simulink model "IRP"  (R2015a)
settings: Solver=ode1  StartTime=0.0  StopTime=Inf  FixedStep=0.001  RelTol=1e-3
PostLoadFcn:
  | , if any(exist('dsrtsu_mdlpostloadfcn', 'file') == [2, 3, 6]), try dsrtsu_mdlpostloadfcn('Execute', bdroot); catch fprintf('Error in PostLoadFcn (dsrtsu_mdlpostloadfcn) for model "%s":\n %s\n', bdroot, lasterr); end, end,
libraries: simulink x8, rtilibm x6, simulink_extras x6
(part 1 of 2)
settings Model: DSRTSU_INTERNAL_RTI_VER=460  DSRTSU_INTERNAL_RTI_TYPE=rti1005  DSRTSU_INTERNAL_RTIFPGA=50  Creator=k19p800a  LastModifiedBy=k19p800a
settings OptimizationCC: BlockReduction=off  OptimizeBlockIOStorage=off  BufferReuse=off  GlobalBufferReuse=off  ExpressionFolding=off  LocalBlockOutputs=off
settings HardwareCC: ProdIntDivRoundTo=Zero  ProdEndianess=BigEndian  ProdHWDeviceType=Generic->Custom  TargetIntDivRoundTo=Zero  TargetEndianess=BigEndian  TargetHWDeviceType=Generic->Custom
settings RTWCC: SystemTargetFile=rti1005.tlc  MakeCommand=make_rti  TemplateMakefile=rti1005.tmf  Description=dSPACE DS1005 Hardware Platform
settings STFCustomTargetCC: GenerateSampleERTMain=off  ParMdlRefBuildCompliant=on  GeneratePreprocessorConditionals=Disable all  ERTCustomFileBanners=off  SupportNonInlinedSFcns=on  SupportVariableSizeSignals=off  MATLABClassNameForMDSCustomization=Simulink.SoftwareTarget.GRTCustomization  GRTInterface=on  SystemTargetFile=rti1005.tlc
settings GRTTargetCC: CompOptLevelCompliant=off  ConcurrentExecutionCompliant=off  CombineOutputUpdateFcns=off  MatFileLogging=off  CPPClassGenCompliant=off  GRTInterface=on  ExtModeMexFile=noextcomm

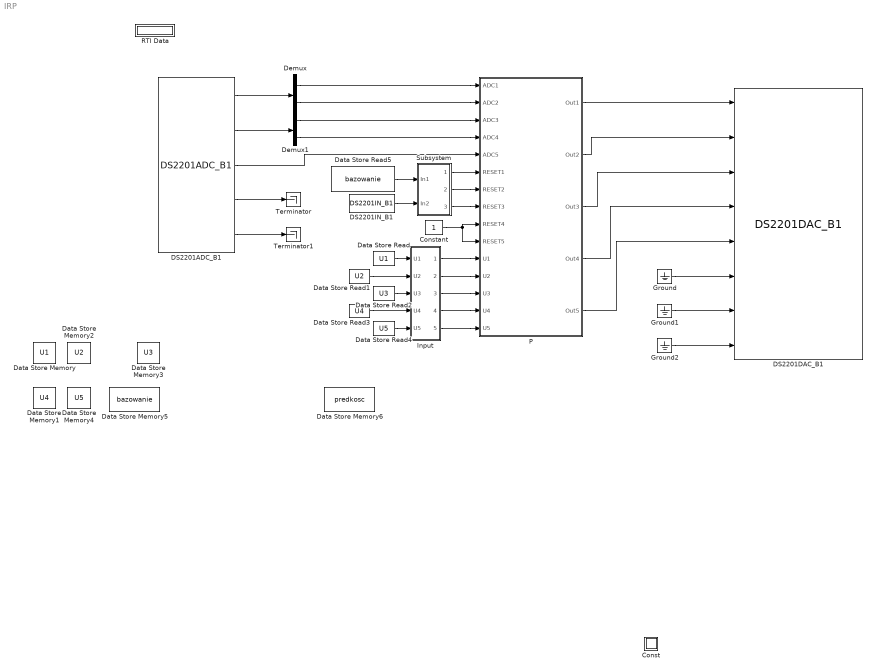
== system IRP ==
  Const : Subsystem
  Constant : Constant
  DS2201ADC_B1 : rtilibm/DS2201/DS2201ADC_B1  BoardNo=1  channelNo1=[1 2 3 4]  channelNo2=[5 6 7 8]  channelNo3=[9 10]  channelNo4=-1  channelNo5=-1  DialogFcn=gui2201adc  UnitName={'DS2201ADC_B'}  UnitValues={ 1 }  DSProperties=struct('RTI',struct('Version',uint32(1),'BlockType',struct('isSLSource',uint8(1),'isSLSink',uint8(0),'isHWSource',uint8(1),'isHWSink',uint8(0),'isSetup',uint8(0),'isInline',uint8(1),'isNonInline',uint8(0),'isInterrupt',uint8(0),'isChannelwise',uint8(0)),'IOBoardType','DS2201','UnitType','ADC','Identifier','ADCMUX','DialogType','ML','BlockSet','NONE','SlaveProcessor','NONE'))
  DS2201DAC_B1 : rtilibm/DS2201/DS2201DAC_B1  BoardNo=1  IOErrorMode=[0 0]  InitValue=[0 0 0 0 0 0 0 0]  TermMode=[1 1 1 1 1 1 1 1]  TermValue=[0 0 0 0 0 0 0 0]  DialogFcn=gui2201dac  UnitName={'DS2201DAC_B'}  UnitValues={ 1 }  DSProperties=struct('RTI',struct('Version',uint32(1),'BlockType',struct('isSLSource',uint8(0),'isSLSink',uint8(1),'isHWSource',uint8(0),'isHWSink',uint8(1),'isSetup',uint8(0),'isInline',uint8(1),'isNonInline',uint8(0),'isInterrupt',uint8(0),'isChannelwise',uint8(0)),'IOBoardType','DS2201','UnitType','DAC','Identifier','DAC','DialogType','ML','BlockSet','NONE','SlaveProcessor','NONE'))
  DS2201IN_B1 : rtilibm/DS2201/DS2201IN_B1  BoardNo=1  ChannelNos=[1 2 3 4 5]  DialogFcn=gui2201in  UnitName={ 'DS2201IN_B' }  UnitValues={ 1 }  DSProperties=struct('RTI',struct('Version',uint32(1),'BlockType',struct('isSLSource',uint8(1),'isSLSink',uint8(0),'isHWSource',uint8(1),'isHWSink',uint8(0),'isSetup',uint8(0),'isInline',uint8(1),'isNonInline',uint8(0),'isInterrupt',uint8(0),'isChannelwise',uint8(0)),'IOBoardType','DS2201','UnitType','BIT','Identifier','BITIN','DialogType','ML','BlockSet','NONE','SlaveProcessor','NONE'))
  Data Store Memory : DataStoreMemory  DataStoreName=U1  ReadBeforeWriteMsg=warning  WriteAfterWriteMsg=warning  WriteAfterReadMsg=warning
  Data Store Memory1 : DataStoreMemory  DataStoreName=U4  ReadBeforeWriteMsg=warning  WriteAfterWriteMsg=warning  WriteAfterReadMsg=warning
  Data Store Memory2 : DataStoreMemory  DataStoreName=U2  ReadBeforeWriteMsg=warning  WriteAfterWriteMsg=warning  WriteAfterReadMsg=warning
  Data Store Memory3 : DataStoreMemory  DataStoreName=U3  ReadBeforeWriteMsg=warning  WriteAfterWriteMsg=warning  WriteAfterReadMsg=warning
  Data Store Memory4 : DataStoreMemory  DataStoreName=U5  ReadBeforeWriteMsg=warning  WriteAfterWriteMsg=warning  WriteAfterReadMsg=warning
  Data Store Memory5 : DataStoreMemory  DataStoreName=bazowanie  ReadBeforeWriteMsg=warning  WriteAfterWriteMsg=warning  WriteAfterReadMsg=warning
  Data Store Memory6 : DataStoreMemory  DataStoreName=predkosc  ReadBeforeWriteMsg=warning  WriteAfterWriteMsg=warning  WriteAfterReadMsg=warning
  Data Store Read : DataStoreRead  DataStoreName=U1
  Data Store Read1 : DataStoreRead  DataStoreName=U2
  Data Store Read2 : DataStoreRead  DataStoreName=U3
  Data Store Read3 : DataStoreRead  DataStoreName=U4
  Data Store Read4 : DataStoreRead  DataStoreName=U5
  Data Store Read5 : DataStoreRead  DataStoreName=bazowanie
  Demux : Demux  Outputs=2
  Demux1 : Demux  Outputs=2
  Ground : Ground
  Ground1 : Ground
  Ground2 : Ground
  Input : Subsystem
  "P " : Subsystem
  RTI Data : Subsystem  Tag=struct('RTIDataServer',struct('RTIDataServerVs','2','RTIModelDescription','struct(''main'',''IRP'',''sub'','''',''isMp'',0)'))  LoadFcn="if exist('rtidc'), try,  rtidc('DataHostBlockClbLoad', gcbh); catch, disp(['Warning: ''LoadFcn'' for RTI Data block failed: ' lasterr]); end, end,"  mask(RTI_DATA_HOST){}
      mask help:
      | RTI Data Block.
      | This block is used by RTI to store internal model-dependent data.
      | Please keep this block on the root level of the model. Deleting this block will result in data loss.
      |
      | NEVER DELETE OR COPY THIS BLOCK!
      settings: CopyFcn="if exist('rtidc'), try,  rtidc('DataHostBlockClbCopy', gcbh); catch, disp(['Warning: ''CopyFcn'' for RTI Data block failed: ' lasterr]); end, end,"  DeleteFcn="if exist('rtidc'), try,  rtidc('DataHostBlockClbDelete', gcbh); catch, disp(['Warning: ''DeleteFcn'' for RTI Data block failed: ' lasterr]); end, end,"  ModelCloseFcn="if exist('rtidc'), try,  rtidc('DataHostBlockClbModelClose', gcbh); catch, disp(['Warning: ''ModelCloseFcn'' for RTI Data block failed: ' lasterr]); end, end,"  PreSaveFcn="if exist('rtidc'), try,  rtidc('DataHostBlockClbPreSave', gcbh); catch, disp(['Warning: ''PreSaveFcn'' for RTI Data block failed: ' lasterr]); end, end,"  PostSaveFcn="if exist('rtidc'), try,  rtidc('DataHostBlockClbPostSave', gcbh); catch, disp(['Warning: ''PostSaveFcn'' for RTI Data block failed: ' lasterr]); end, end,"  NameChangeFcn="if exist('rtidc'), try,  rtidc('DataHostBlockClbNameChange', gcbh); catch, disp(['Warning: ''NameChangeFcn'' for RTI Data block failed: ' lasterr]); end, end,"
      mask Help:
      | RTI Data Block.
      | This block is used by RTI to store internal model-dependent data.
      | Please keep this block on the root level of the model. Deleting this block will result in data loss.
      | 
      | NEVER DELETE OR COPY THIS BLOCK!
      mask Display:
      | text(0.5, 0.5, 'RTI Data', 'HorizontalAlignment', 'center');
      | plot([1 0]);
  Subsystem : Subsystem
  Terminator : Terminator
  Terminator1 : Terminator
  wires:
  DS2201ADC_B1/1 -> Demux/1
  DS2201ADC_B1/2 -> Demux1/1
  DS2201ADC_B1/4 -> Terminator/1
  DS2201ADC_B1/5 -> Terminator1/1
  Demux/1 -> "P "/1("ADC1 ")
  Demux/2 -> "P "/2(ADC2)
  Demux1/1 -> "P "/3(ADC3)
  Demux1/2 -> "P "/4(ADC4)
  DS2201ADC_B1/3 -> "P "/5(ADC5)
  "P "/1(Out1) -> DS2201DAC_B1/1
  "P "/2(Out2) -> DS2201DAC_B1/2
  "P "/3(Out3) -> DS2201DAC_B1/3
  "P "/4(Out4) -> DS2201DAC_B1/4
  "P "/5(Out5) -> DS2201DAC_B1/5
  Ground/1 -> DS2201DAC_B1/6
  Ground1/1 -> DS2201DAC_B1/7
  Ground2/1 -> DS2201DAC_B1/8
  Input/1(Out1) -> "P "/11(U1)
  Input/2(Out2) -> "P "/12(U2)
  Input/3(Out3) -> "P "/13(U3)
  Input/4(Out4) -> "P "/14(U4)
  Input/5(Out5) -> "P "/15(U5)
  Data Store Read/1 -> Input/1(U1)
  Data Store Read1/1 -> Input/2(U2)
  Data Store Read2/1 -> Input/3(U3)
  Data Store Read3/1 -> Input/4(U4)
  Data Store Read4/1 -> Input/5(U5)
  Data Store Read5/1 -> Subsystem/1(In1)
  DS2201IN_B1/1 -> Subsystem/2(In2)
  Subsystem/1(Res1) -> "P "/6(RESET1)
  Subsystem/2(Res2) -> "P "/7(RESET2)
  Subsystem/3(Res3) -> "P "/8(RESET3)
  Constant/1 -> "P "/10(RESET5), "P "/9(RESET4)

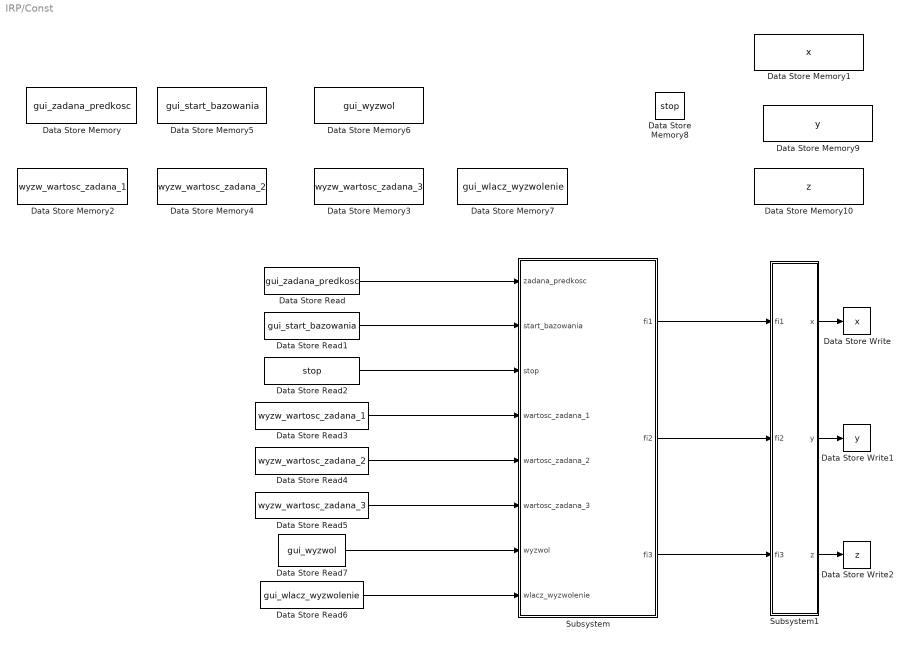
== system IRP/Const ==
  Data Store Memory : DataStoreMemory  DataStoreName=gui_zadana_predkosc  ReadBeforeWriteMsg=warning  WriteAfterWriteMsg=warning  WriteAfterReadMsg=warning  InitialValue=100
  Data Store Memory1 : DataStoreMemory  DataStoreName=x  ReadBeforeWriteMsg=warning  WriteAfterWriteMsg=warning  WriteAfterReadMsg=warning
  Data Store Memory10 : DataStoreMemory  DataStoreName=z  ReadBeforeWriteMsg=warning  WriteAfterWriteMsg=warning  WriteAfterReadMsg=warning
  Data Store Memory2 : DataStoreMemory  DataStoreName=wyzw_wartosc_zadana_1  ReadBeforeWriteMsg=warning  WriteAfterWriteMsg=warning  WriteAfterReadMsg=warning
  Data Store Memory3 : DataStoreMemory  DataStoreName=wyzw_wartosc_zadana_3  ReadBeforeWriteMsg=warning  WriteAfterWriteMsg=warning  WriteAfterReadMsg=warning
  Data Store Memory4 : DataStoreMemory  DataStoreName=wyzw_wartosc_zadana_2  ReadBeforeWriteMsg=warning  WriteAfterWriteMsg=warning  WriteAfterReadMsg=warning
  Data Store Memory5 : DataStoreMemory  DataStoreName=gui_start_bazowania  ReadBeforeWriteMsg=warning  WriteAfterWriteMsg=warning  WriteAfterReadMsg=warning
  Data Store Memory6 : DataStoreMemory  DataStoreName=gui_wyzwol  ReadBeforeWriteMsg=warning  WriteAfterWriteMsg=warning  WriteAfterReadMsg=warning
  Data Store Memory7 : DataStoreMemory  DataStoreName=gui_wlacz_wyzwolenie  ReadBeforeWriteMsg=warning  WriteAfterWriteMsg=warning  WriteAfterReadMsg=warning
  Data Store Memory8 : DataStoreMemory  DataStoreName=stop  ReadBeforeWriteMsg=warning  WriteAfterWriteMsg=warning  WriteAfterReadMsg=warning
  Data Store Memory9 : DataStoreMemory  DataStoreName=y  ReadBeforeWriteMsg=warning  WriteAfterWriteMsg=warning  WriteAfterReadMsg=warning
  Data Store Read : DataStoreRead  DataStoreName=gui_zadana_predkosc
  Data Store Read1 : DataStoreRead  DataStoreName=gui_start_bazowania
  Data Store Read2 : DataStoreRead  DataStoreName=stop
  Data Store Read3 : DataStoreRead  DataStoreName=wyzw_wartosc_zadana_1
  Data Store Read4 : DataStoreRead  DataStoreName=wyzw_wartosc_zadana_2
  Data Store Read5 : DataStoreRead  DataStoreName=wyzw_wartosc_zadana_3
  Data Store Read6 : DataStoreRead  DataStoreName=gui_wlacz_wyzwolenie
  Data Store Read7 : DataStoreRead  DataStoreName=gui_wyzwol
  Data Store Write : DataStoreWrite  DataStoreName=x
  Data Store Write1 : DataStoreWrite  DataStoreName=y
  Data Store Write2 : DataStoreWrite  DataStoreName=z
  Subsystem : Subsystem
  Subsystem1 : Subsystem
  wires:
  Data Store Read/1 -> Subsystem/1("zadana_predkosc ")
  Data Store Read1/1 -> Subsystem/2(start_bazowania)
  Data Store Read2/1 -> Subsystem/3(stop)
  Data Store Read3/1 -> Subsystem/4(wartosc_zadana_1)
  Data Store Read4/1 -> Subsystem/5(wartosc_zadana_2)
  Data Store Read5/1 -> Subsystem/6(wartosc_zadana_3)
  Data Store Read7/1 -> Subsystem/7(wyzwol)
  Data Store Read6/1 -> Subsystem/8("wlacz_wyzwolenie ")
  Subsystem/1(fi1) -> Subsystem1/1(fi1)
  Subsystem/2(fi2) -> Subsystem1/2(fi2)
  Subsystem/3(fi3) -> Subsystem1/3(fi3)
  Subsystem1/1(x) -> Data Store Write/1
  Subsystem1/2(y) -> Data Store Write1/1
  Subsystem1/3(z) -> Data Store Write2/1

== system IRP/Input ==
  U1 : Inport
  U2 : Inport  Port=2
  U3 : Inport  Port=3
  U4 : Inport  Port=4
  U5 : Inport  Port=5
  Demux : Demux  Outputs=5
  "Logic " : Subsystem
  Memory : Memory
  Mux : Mux  Inputs=5
  Switch : Switch  Criteria=u2 > Threshold
  Out1 : Outport
  Out2 : Outport  Port=2
  Out3 : Outport  Port=3
  Out4 : Outport  Port=4
  Out5 : Outport  Port=5
  wires:
  Mux/1 -> Switch/1
  U2/1 -> "Logic "/2(In2), Mux/2
  U3/1 -> "Logic "/3(In3), Mux/3
  U4/1 -> "Logic "/4(In4), Mux/4
  U5/1 -> "Logic "/5(In5), Mux/5
  Demux/1 -> Out1/1
  Demux/2 -> Out2/1
  Demux/3 -> Out3/1
  Demux/4 -> Out4/1
  Demux/5 -> Out5/1
  Switch/1 -> Memory/1, Demux/1
  U1/1 -> "Logic "/1(In1), Mux/1
  "Logic "/1(Out1) -> Switch/2
  Memory/1 -> Switch/3

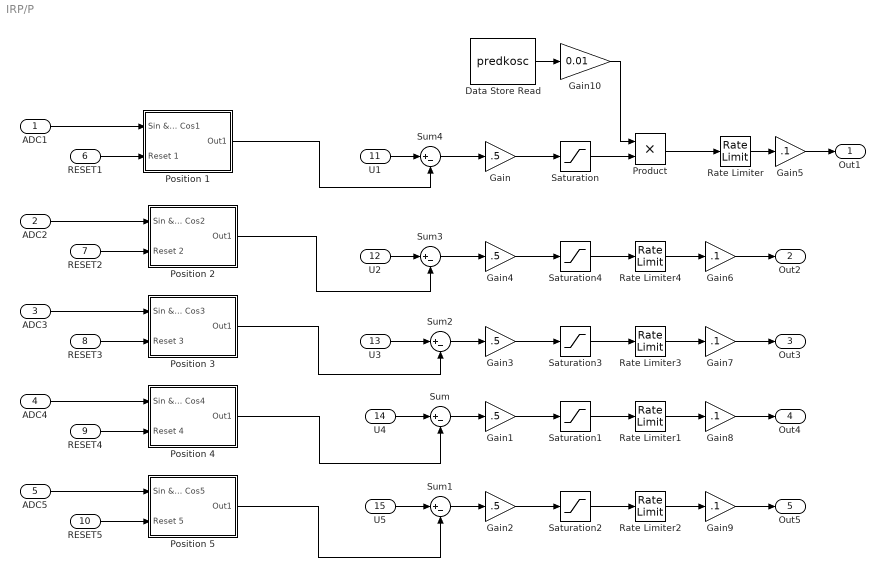
== system IRP/P  ==
  "ADC1 " : Inport
  ADC2 : Inport  Port=2
  ADC3 : Inport  Port=3
  ADC4 : Inport  Port=4
  ADC5 : Inport  Port=5
  RESET1 : Inport  Port=6
  RESET2 : Inport  Port=7
  RESET3 : Inport  Port=8
  RESET4 : Inport  Port=9
  RESET5 : Inport  Port=10
  U1 : Inport  Port=11
  U2 : Inport  Port=12
  U3 : Inport  Port=13
  U4 : Inport  Port=14
  U5 : Inport  Port=15
  Data Store Read : DataStoreRead  DataStoreName=predkosc
  Gain{,1..4} (5 alike) : Gain  Gain=.5
  Gain10 : Gain  Gain=0.01
  Gain{5..9} (5 alike) : Gain  Gain=.1
  Position 1 : Subsystem
  Position 2 : Subsystem
  Position 3 : Subsystem
  Position 4 : Subsystem
  Position 5 : Subsystem
  Product : Product
  Rate Limiter{,1..4} (5 alike) : RateLimiter  RisingSlewLimit=50  FallingSlewLimit=-50  SampleTimeMode=inherited
  Saturation{,1..4} (5 alike) : Saturate  UpperLimit=3  LowerLimit=-3
  Sum{,1..4} (5 alike) : Sum  Inputs=|+-
  Out1 : Outport
  Out2 : Outport  Port=2
  Out3 : Outport  Port=3
  Out4 : Outport  Port=4
  Out5 : Outport  Port=5
  wires:
  Gain3/1 -> Saturation3/1
  Saturation4/1 -> Rate Limiter4/1
  Saturation3/1 -> Rate Limiter3/1
  Rate Limiter4/1 -> Gain6/1
  Rate Limiter2/1 -> Gain9/1
  Gain4/1 -> Saturation4/1
  Rate Limiter3/1 -> Gain7/1
  Rate Limiter1/1 -> Gain8/1
  Gain2/1 -> Saturation2/1
  Saturation1/1 -> Rate Limiter1/1
  Gain1/1 -> Saturation1/1
  Rate Limiter/1 -> Gain5/1
  Saturation2/1 -> Rate Limiter2/1
  Sum1/1 -> Gain2/1
  Sum2/1 -> Gain3/1
  Sum3/1 -> Gain4/1
  Sum4/1 -> Gain/1
  Sum/1 -> Gain1/1
  Gain5/1 -> Out1/1
  Gain6/1 -> Out2/1
  Gain7/1 -> Out3/1
  Gain8/1 -> Out4/1
  Gain9/1 -> Out5/1
  Position 1/1(Out1) -> Sum4/2
  ADC2/1 -> Position 2/1(Sin && Cos2)
  Position 2/1(Out1) -> Sum3/2
  ADC3/1 -> Position 3/1(Sin && Cos3)
  ADC4/1 -> Position 4/1(Sin && Cos4)
  Position 4/1(Out1) -> Sum/2
  ADC5/1 -> Position 5/1(Sin && Cos5)
  Position 5/1(Out1) -> Sum1/2
  Position 3/1(Out1) -> Sum2/2
  "ADC1 "/1 -> Position 1/1(Sin && Cos1)
  RESET1/1 -> Position 1/2(Reset 1)
  RESET2/1 -> Position 2/2(Reset 2)
  RESET3/1 -> Position 3/2(Reset 3)
  RESET4/1 -> Position 4/2(Reset 4)
  RESET5/1 -> Position 5/2(Reset 5)
  U1/1 -> Sum4/1
  U2/1 -> Sum3/1
  U3/1 -> Sum2/1
  U4/1 -> Sum/1
  U5/1 -> Sum1/1
  Gain10/1 -> Product/1
  Gain/1 -> Saturation/1
  Saturation/1 -> Product/2
  Product/1 -> Rate Limiter/1
  Data Store Read/1 -> Gain10/1

== system IRP/RTI Data ==
  RTI Data Store : Subsystem  Tag="struct('private',struct('version',struct('dsVer',uint32(2),'dsVerCreation',uint32(2),'RTI',struct('ver','7.4','type','RTI1005')),'access',struct('type','Model','isPerm',1,'created',['11-Mar-2019 08:34:42'],'modified',['18-Mar-2019 09:25:52'],'location','')),'public',struct('main',struct('data',[]),'sub',struct('name',{{'IRP'}},'data',{{struct('TH',struct('thTaskInfo',struct('taskType',{'TIMER','HWINT','TMRINT','SWINT','GLINT'},'tasksNumOf',{1,0,0,0,0},'srcIds',{{'TIMERA'},{},{},{},{}},'taskNames',{{['Timer Task 1']},{},{},{},{}})),'th_tc',struct('dataType','TASK','taskGroupId','','taskGroupList',{{}},'taskSchedulingPolicy','FCFS','taskType','TIMER','blkh',-1,'srcId','TIMERA','srcSgnName',['Timer A interrupt'],'srcCpuName','','taskName',['Timer Task 1  [0.001] s'],'taskNameDisplayExt','','smplTime',0.001,'smplTimeOffs',0,'hasFixedPriority',0,'priority',1,'hasFixedOvc',0,'ovcType',1,'ovcMax',1),'tc_th',struct('dataType','TASK','taskGroupId','','taskGroupList',{{}},'taskSchedulingPolicy','FCFS','taskType','TIMER','blkh',-1,'srcId','TIMERA','srcSgnName',['Timer A interrupt'],'srcCpuName','','taskName',['Timer Task 1  [0.001] s'],'taskNameDisplayExt','','smplTime',0.001,'smplTimeOffs',0,'hasFixedPriority',0,'priority',1,'hasFixedOvc',0,'ovcType',1,'ovcMax',1))}})))"  mask(RTI_DATA_STORE){}
      mask help:
      | RTI Data Store Block. This block is used by RTI to store internal model dependent data. Deleting this block will result in data loss.
      |
      | NEVER DELETE, COPY, OR MODIFY THIS BLOCK!
      mask Help:
      | RTI Data Store Block. This block is used by RTI to store internal model dependent data. Deleting this block will result in data loss.
      | 
      | NEVER DELETE, COPY, OR MODIFY THIS BLOCK!
      mask Display: text(0.5, 0.5, ' ', 'HorizontalAlignment', 'center');

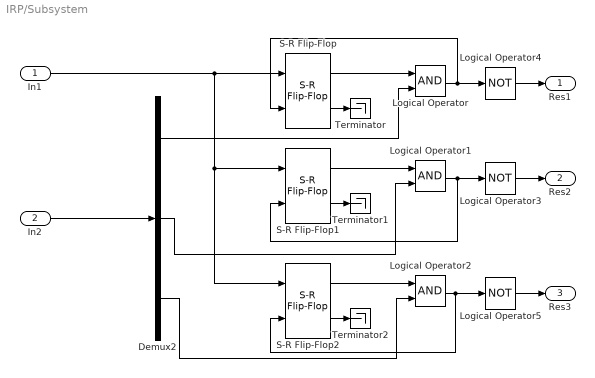
== system IRP/Subsystem ==
  In1 : Inport
  In2 : Inport  Port=2
  Demux2 : Demux  Outputs=3
  Logical Operator : Logic  AllPortsSameDT=off
  Logical Operator1 : Logic  AllPortsSameDT=off
  Logical Operator2 : Logic  AllPortsSameDT=off
  Logical Operator3 : Logic  Operator=NOT  AllPortsSameDT=off
  Logical Operator4 : Logic  Operator=NOT  AllPortsSameDT=off
  Logical Operator5 : Logic  Operator=NOT  AllPortsSameDT=off
  S-R Flip-Flop : simulink_extras/Flip Flops/S-R Flip-Flop  initial_condition=0
  S-R Flip-Flop1 : simulink_extras/Flip Flops/S-R Flip-Flop  initial_condition=0
  S-R Flip-Flop2 : simulink_extras/Flip Flops/S-R Flip-Flop  initial_condition=0
  Terminator : Terminator
  Terminator1 : Terminator
  Terminator2 : Terminator
  Res1 : Outport
  Res2 : Outport  Port=2
  Res3 : Outport  Port=3
  wires:
  Logical Operator1/1 -> Logical Operator3/1, S-R Flip-Flop1/2
  In1/1 -> S-R Flip-Flop1/1, S-R Flip-Flop2/1, S-R Flip-Flop/1
  In2/1 -> Demux2/1
  S-R Flip-Flop/1 -> Logical Operator/1
  Demux2/1 -> Logical Operator/2
  Logical Operator/1 -> S-R Flip-Flop/2, Logical Operator4/1
  Demux2/3 -> Logical Operator2/2
  S-R Flip-Flop2/1 -> Logical Operator2/1
  Demux2/2 -> Logical Operator1/2
  S-R Flip-Flop1/1 -> Logical Operator1/1
  Logical Operator2/1 -> Logical Operator5/1, S-R Flip-Flop2/2
  S-R Flip-Flop/2 -> Terminator/1
  S-R Flip-Flop2/2 -> Terminator2/1
  S-R Flip-Flop1/2 -> Terminator1/1
  Logical Operator4/1 -> Res1/1
  Logical Operator3/1 -> Res2/1
  Logical Operator5/1 -> Res3/1

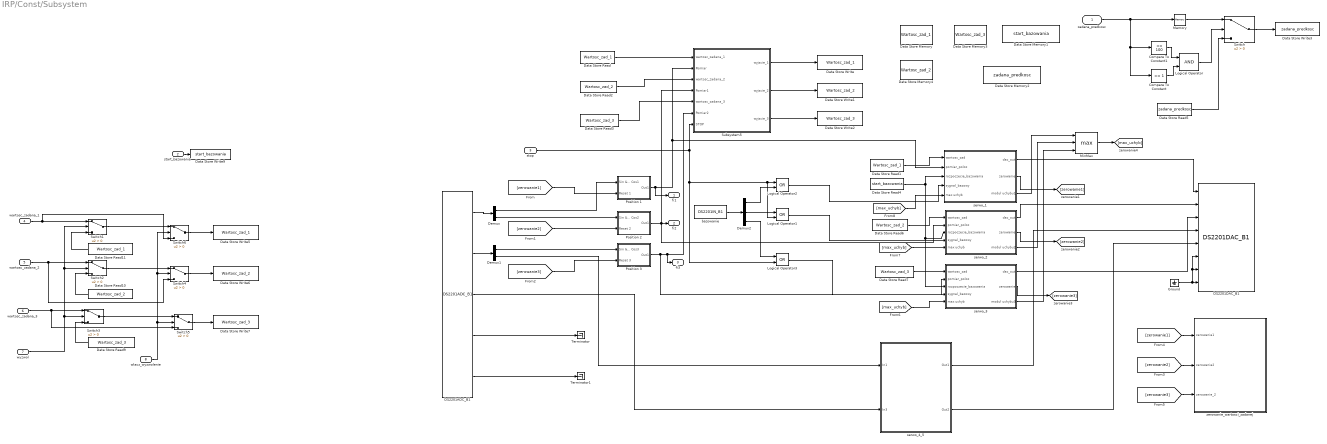
== system IRP/Const/Subsystem ==
  "zadana_predkosc " : Inport
  start_bazowania : Inport  Port=2
  stop : Inport  Port=3
  wartosc_zadana_1 : Inport  Port=4
  wartosc_zadana_2 : Inport  Port=5
  wartosc_zadana_3 : Inport  Port=6
  wyzwol : Inport  Port=7
  "wlacz_wyzwolenie " : Inport  Port=8
  Compare To Constant : simulink/Logic and Bit Operations/Compare To Constant  relop=>=  const=1  OutDataTypeStr=boolean
  Compare To Constant1 : simulink/Logic and Bit Operations/Compare To Constant  relop=<=  const=100  OutDataTypeStr=boolean
  DS2201ADC_B1 : rtilibm/DS2201/DS2201ADC_B1  BoardNo=1  channelNo1=[1 2 3 4]  channelNo2=[5 6 7 8]  channelNo3=[9 10]  channelNo4=-1  channelNo5=-1  DialogFcn=gui2201adc  UnitName={'DS2201ADC_B'}  UnitValues={ 1 }  DSProperties=struct('RTI',struct('Version',uint32(1),'BlockType',struct('isSLSource',uint8(1),'isSLSink',uint8(0),'isHWSource',uint8(1),'isHWSink',uint8(0),'isSetup',uint8(0),'isInline',uint8(1),'isNonInline',uint8(0),'isInterrupt',uint8(0),'isChannelwise',uint8(0)),'IOBoardType','DS2201','UnitType','ADC','Identifier','ADCMUX','DialogType','ML','BlockSet','NONE','SlaveProcessor','NONE'))
  DS2201DAC_B1 : rtilibm/DS2201/DS2201DAC_B1  BoardNo=1  IOErrorMode=[0 0]  InitValue=[0 0 0 0 0 0 0 0]  TermMode=[0 0 0 0 0 0 0 0]  TermValue=[0 0 0 0 0 0 0 0]  DialogFcn=gui2201dac  UnitName={'DS2201DAC_B'}  UnitValues={ 1 }  DSProperties=struct('RTI',struct('Version',uint32(1),'BlockType',struct('isSLSource',uint8(0),'isSLSink',uint8(1),'isHWSource',uint8(0),'isHWSink',uint8(1),'isSetup',uint8(0),'isInline',uint8(1),'isNonInline',uint8(0),'isInterrupt',uint8(0),'isChannelwise',uint8(0)),'IOBoardType','DS2201','UnitType','DAC','Identifier','DAC','DialogType','ML','BlockSet','NONE','SlaveProcessor','NONE'))
  Data Store Memory : DataStoreMemory  DataStoreName=Wartosc_zad_1  ReadBeforeWriteMsg=warning  WriteAfterWriteMsg=warning  WriteAfterReadMsg=warning
  Data Store Memory1 : DataStoreMemory  DataStoreName=start_bazowania  ReadBeforeWriteMsg=warning  WriteAfterWriteMsg=warning  WriteAfterReadMsg=warning
  Data Store Memory2 : DataStoreMemory  DataStoreName=zadana_predkosc  ReadBeforeWriteMsg=warning  WriteAfterWriteMsg=warning  WriteAfterReadMsg=warning
  Data Store Memory3 : DataStoreMemory  DataStoreName=Wartosc_zad_3  ReadBeforeWriteMsg=warning  WriteAfterWriteMsg=warning  WriteAfterReadMsg=warning
  Data Store Memory4 : DataStoreMemory  DataStoreName=Wartosc_zad_2  ReadBeforeWriteMsg=warning  WriteAfterWriteMsg=warning  WriteAfterReadMsg=warning
  Data Store Read : DataStoreRead  DataStoreName=Wartosc_zad_1
  Data Store Read1 : DataStoreRead  DataStoreName=Wartosc_zad_1
  Data Store Read10 : DataStoreRead  DataStoreName=Wartosc_zad_2
  Data Store Read11 : DataStoreRead  DataStoreName=Wartosc_zad_1
  Data Store Read2 : DataStoreRead  DataStoreName=Wartosc_zad_2
  Data Store Read3 : DataStoreRead  DataStoreName=Wartosc_zad_3
  Data Store Read4 : DataStoreRead  DataStoreName=start_bazowania
  Data Store Read5 : DataStoreRead  DataStoreName=zadana_predkosc
  Data Store Read6 : DataStoreRead  DataStoreName=Wartosc_zad_2
  Data Store Read7 : DataStoreRead  DataStoreName=Wartosc_zad_3
  Data Store Read9 : DataStoreRead  DataStoreName=Wartosc_zad_3
  Data Store Write : DataStoreWrite  DataStoreName=Wartosc_zad_1
  Data Store Write1 : DataStoreWrite  DataStoreName=Wartosc_zad_2
  Data Store Write2 : DataStoreWrite  DataStoreName=Wartosc_zad_3
  Data Store Write3 : DataStoreWrite  DataStoreName=zadana_predkosc
  Data Store Write5 : DataStoreWrite  DataStoreName=Wartosc_zad_1
  Data Store Write6 : DataStoreWrite  DataStoreName=Wartosc_zad_2
  Data Store Write7 : DataStoreWrite  DataStoreName=Wartosc_zad_3
  Data Store Write9 : DataStoreWrite  DataStoreName=start_bazowania
  Demux : Demux  Outputs=2
  Demux1 : Demux  Outputs=2
  Demux2 : Demux  Outputs=3
  Ground : Ground
  Logical Operator : Logic  AllPortsSameDT=off  OutDataTypeStr=boolean
  Logical Operator1 : Logic  Operator=OR  AllPortsSameDT=off
  Logical Operator2 : Logic  Operator=OR  AllPortsSameDT=off
  Logical Operator3 : Logic  Operator=OR  AllPortsSameDT=off
  Memory : Memory
  MinMax : MinMax  Function=max  Inputs=3
  Position 1 : Subsystem
  Position 2 : Subsystem
  Position 3 : Subsystem
  Subsystem5 : Subsystem
  Switch{,1..6} (7 alike) : Switch  Criteria=u2 > Threshold
  Terminator : Terminator
  Terminator1 : Terminator
  bazowanie : rtilibm/DS2201/DS2201IN_B1  BoardNo=1  ChannelNos=[1 2 3]  DialogFcn=gui2201in  UnitName={ 'DS2201IN_B' }  UnitValues={ 1 }  DSProperties=struct('RTI',struct('Version',uint32(1),'BlockType',struct('isSLSource',uint8(1),'isSLSink',uint8(0),'isHWSource',uint8(1),'isHWSink',uint8(0),'isSetup',uint8(0),'isInline',uint8(1),'isNonInline',uint8(0),'isInterrupt',uint8(0),'isChannelwise',uint8(0)),'IOBoardType','DS2201','UnitType','BIT','Identifier','BITIN','DialogType','ML','BlockSet','NONE','SlaveProcessor','NONE'))
  serwo_1 : Subsystem
  serwo_2 : Subsystem
  serwo_3 : Subsystem
  serwo_4_5 : Subsystem
  zerowanie_wartosci_zadanej : Subsystem
  fi1 : Outport
  fi2 : Outport  Port=2
  fi3 : Outport  Port=3
  wires:
  serwo_2/3(moduł uchybu2) -> MinMax/2
  serwo_1/3(moduł uchybu1) -> MinMax/1
  serwo_3/3(moduł uchybu3) -> MinMax/3
  start_bazowania/1 -> Data Store Write9/1
  Switch/1 -> Data Store Write3/1
  Logical Operator/1 -> Switch/2
  "zadana_predkosc "/1 -> Compare To Constant/1, Compare To Constant1/1, Memory/1
  Data Store Read5/1 -> Switch/3
  MinMax/1 -> [max_uchyb]
  [max_uchyb] -> serwo_2/5(max uchyb)
  [max_uchyb] -> serwo_1/5(max uchyb)
  [max_uchyb] -> serwo_3/5(max uchyb)
  DS2201ADC_B1/1 -> Demux/1
  DS2201ADC_B1/2 -> Demux1/1
  DS2201ADC_B1/5 -> Terminator1/1
  DS2201ADC_B1/4 -> Terminator/1
  Demux/1 -> Position 1/1(Sin && Cos1)
  Demux/2 -> Position 2/1(Sin && Cos2)
  Demux1/1 -> Position 3/1(Sin && Cos3)
  serwo_1/1(dac_out) -> DS2201DAC_B1/1
  serwo_2/1(dac_out) -> DS2201DAC_B1/2
  serwo_3/1(dac_out) -> DS2201DAC_B1/3
  Ground/1 -> DS2201DAC_B1/6, DS2201DAC_B1/7, DS2201DAC_B1/8
  Data Store Read/1 -> Subsystem5/1(wartosc_zadana_1)
  Position 1/1(Out1) -> Subsystem5/2(Pomiar), serwo_1/2(pomiar_poloz), fi1/1
  Data Store Read2/1 -> Subsystem5/3(wartosc_zadana_2)
  Position 2/1(Out1) -> fi2/1, serwo_2/2(pomiar_poloz), Subsystem5/4(Pomiar1)
  Data Store Read3/1 -> Subsystem5/5(wartosc_zadana_3)
  Position 3/1(Out1) -> serwo_3/2(pomiar_poloz), fi3/1, Subsystem5/6(Pomiar2)
  Subsystem5/1(wyjscie_1) -> Data Store Write/1
  Subsystem5/2(wyjscie_2) -> Data Store Write1/1
  Subsystem5/3("wyjscie_3 ") -> Data Store Write2/1
  Data Store Read1/1 -> serwo_1/1(wartosc_zad)
  Data Store Read6/1 -> serwo_2/1(wartosc_zad)
  Data Store Read7/1 -> serwo_3/1(wartosc_zad)
  stop/1 -> Subsystem5/7(STOP), Logical Operator3/2, Logical Operator1/2, Logical Operator2/1
  Demux1/2 -> serwo_4_5/1(In1)
  DS2201ADC_B1/3 -> serwo_4_5/2(In3)
  serwo_4_5/1(Out1) -> DS2201DAC_B1/4
  serwo_4_5/2(Out2) -> DS2201DAC_B1/5
  Data Store Read4/1 -> serwo_3/3(rozpoczecie_bazowania), serwo_2/3(rozpoczecie_bazowania), serwo_1/3(rozpoczecie_bazowania)
  bazowanie/1 -> Demux2/1
  Demux2/1 -> Logical Operator2/2
  Demux2/2 -> Logical Operator1/1
  Demux2/3 -> Logical Operator3/1
  Logical Operator2/1 -> serwo_1/4(sygnal_bazowy)
  Logical Operator1/1 -> serwo_2/4(sygnal_bazowy)
  Logical Operator3/1 -> serwo_3/4(sygnal_bazowy)
  serwo_1/2(zerowanie) -> [zerowanie1]
  serwo_2/2(zerowanie) -> [zerowanie2]
  serwo_3/2(zerowanie) -> [zerowanie3]
  [zerowanie1] -> Position 1/2(Reset 1)
  [zerowanie2] -> Position 2/2(Reset 2)
  [zerowanie3] -> Position 3/2(Reset 3)
  [zerowanie1] -> zerowanie_wartosci_zadanej/1(zerowanie1)
  [zerowanie2] -> zerowanie_wartosci_zadanej/2(zerowanie2)
  [zerowanie3] -> zerowanie_wartosci_zadanej/3(zerowanie_2)
  Compare To Constant1/1 -> Logical Operator/1
  Compare To Constant/1 -> Logical Operator/2
  wartosc_zadana_1/1 -> Switch6/3, Switch1/1
  wyzwol/1 -> Switch3/2, Switch2/2, Switch1/2
  wartosc_zadana_2/1 -> Switch4/3, Switch2/1
  wartosc_zadana_3/1 -> Switch5/3, Switch3/1
  Data Store Read9/1 -> Switch3/3
  Data Store Read10/1 -> Switch2/3
  Data Store Read11/1 -> Switch1/3
  Switch1/1 -> Switch6/1
  Switch2/1 -> Switch4/1
  Switch3/1 -> Switch5/1
  "wlacz_wyzwolenie "/1 -> Switch5/2, Switch4/2, Switch6/2
  Switch5/1 -> Data Store Write7/1
  Switch4/1 -> Data Store Write6/1
  Switch6/1 -> Data Store Write5/1
  Memory/1 -> Switch/1

== system IRP/Const/Subsystem1 ==
  fi1 : Inport
  fi2 : Inport  Port=2
  fi3 : Inport  Port=3
  Gain : Gain  Gain=pi/180
  Gain1 : Gain  Gain=pi/180
  Gain2 : Gain  Gain=pi/180
  Subsystem : Subsystem
  Subsystem1 : Subsystem
  Subsystem2 : Subsystem
  p1 : Constant  Value=700
  p2 : Constant  Value=450
  p3 : Constant  Value=670
  x : Outport
  y : Outport  Port=2
  z : Outport  Port=3
  wires:
  Subsystem1/1(y) -> y/1
  fi1/1 -> Gain/1
  Subsystem/1(x) -> x/1
  Gain/1 -> Subsystem1/1(fi1), Subsystem/1(fi1)
  fi2/1 -> Gain1/1
  fi3/1 -> Gain2/1
  p1/1 -> Subsystem2/1(p1)
  Gain1/1 -> Subsystem1/2(fi2), Subsystem/2(fi2), Subsystem2/2(fi2)
  Gain2/1 -> Subsystem/3(fi3), Subsystem1/3(fi3), Subsystem2/3(fi3)
  p2/1 -> Subsystem2/4(p2), Subsystem1/4(p2), Subsystem/4(p2)
  p3/1 -> Subsystem2/5(p3), Subsystem1/5(p3), Subsystem/5(p3)
  Subsystem2/1(z) -> z/1

== system IRP/Input/Logic  ==
  In1 : Inport
  In2 : Inport  Port=2
  In3 : Inport  Port=3
  In4 : Inport  Port=4
  In5 : Inport  Port=5
  Logical Operator : Logic  Operator=NOR  Inputs=5  AllPortsSameDT=off
  Subsystem : Subsystem
  Subsystem1 : Subsystem
  Subsystem2 : Subsystem
  Subsystem3 : Subsystem
  Subsystem4 : Subsystem
  Out1 : Outport
  wires:
  Subsystem/1(Out1) -> Logical Operator/1
  Subsystem2/1(Out1) -> Logical Operator/3
  Subsystem1/1(Out1) -> Logical Operator/2
  In2/1 -> Subsystem1/1(In1)
  Subsystem4/1(Out1) -> Logical Operator/5
  In1/1 -> Subsystem/1(In1)
  In4/1 -> Subsystem3/1(In1)
  Logical Operator/1 -> Out1/1
  Subsystem3/1(Out1) -> Logical Operator/4
  In3/1 -> Subsystem2/1(In1)
  In5/1 -> Subsystem4/1(In1)

== system IRP/P /Position 1 ==
  Sin && Cos1 : Inport
  Reset 1 : Inport  Port=2
  Filters 1 : Subsystem
  Position Calculation 1 : Subsystem
  Out1 : Outport
  wires:
  Position Calculation 1/1(Position) -> Out1/1
  Reset 1/1 -> Position Calculation 1/3(Reset (Impulse))
  Sin && Cos1/1 -> Filters 1/1(Sin && Cos)
  Filters 1/2(Cos) -> Position Calculation 1/2(Cos)
  Filters 1/1(Sin) -> Position Calculation 1/1(Sin)

== system IRP/P /Position 2 ==
  Sin && Cos2 : Inport
  Reset 2 : Inport  Port=2
  Filters 2 : Subsystem
  Position Calculation 2 : Subsystem
  Out1 : Outport
  wires:
  Position Calculation 2/1(Position) -> Out1/1
  Reset 2/1 -> Position Calculation 2/3(Reset (Impulse))
  Sin && Cos2/1 -> Filters 2/1(Sin && Cos)
  Filters 2/2(Cos) -> Position Calculation 2/2(Cos)
  Filters 2/1(Sin) -> Position Calculation 2/1(Sin)

== system IRP/P /Position 3 ==
  Sin && Cos3 : Inport
  Reset 3 : Inport  Port=2
  Filters 3 : Subsystem
  Position Calculation 3 : Subsystem
  Out1 : Outport
  wires:
  Position Calculation 3/1(Position) -> Out1/1
  Reset 3/1 -> Position Calculation 3/3(Reset (Impulse))
  Sin && Cos3/1 -> Filters 3/1(Sin && Cos)
  Filters 3/2(Cos) -> Position Calculation 3/2(Cos)
  Filters 3/1(Sin) -> Position Calculation 3/1(Sin)

== system IRP/P /Position 4 ==
  Sin && Cos4 : Inport
  Reset 4 : Inport  Port=2
  Filters 4 : Subsystem
  Position Calculation 4 : Subsystem
  Out1 : Outport
  wires:
  Filters 4/1(Sin) -> Position Calculation 4/1(Sin)
  Filters 4/2(Cos) -> Position Calculation 4/2(Cos)
  Sin && Cos4/1 -> Filters 4/1(Sin && Cos)
  Reset 4/1 -> Position Calculation 4/3(Reset (Impulse))
  Position Calculation 4/1(Position) -> Out1/1

== system IRP/P /Position 5 ==
  Sin && Cos5 : Inport
  Reset 5 : Inport  Port=2
  Filters 5 : Subsystem
  Position Calculation 5 : Subsystem
  Out1 : Outport
  wires:
  Filters 5/1(Sin) -> Position Calculation 5/1(Sin)
  Filters 5/2(Cos) -> Position Calculation 5/2(Cos)
  Sin && Cos5/1 -> Filters 5/1(Sin && Cos)
  Reset 5/1 -> Position Calculation 5/3(Reset (Impulse))
  Position Calculation 5/1(Position) -> Out1/1

== system IRP/RTI Data/RTI Data Store ==
  RTI Data Store : Subsystem  mask(RTI_DATA_STORE){}
      mask help:
      | RTI Data Store Block. This block is used by RTI to store internal model dependent data. Deleting this block will result in data loss.
      |
      | NEVER DELETE, COPY, OR MODIFY THIS BLOCK!
      mask Help:
      | RTI Data Store Block. This block is used by RTI to store internal model dependent data. Deleting this block will result in data loss.
      | 
      | NEVER DELETE, COPY, OR MODIFY THIS BLOCK!
      mask Display: text(0.5, 0.5, ' ', 'HorizontalAlignment', 'center');

== system IRP/Const/Subsystem/Position 1 ==
  Sin && Cos1 : Inport
  Reset 1 : Inport  Port=2
  Filters 1 : Subsystem
  Position Calculation 1 : Subsystem
  Out1 : Outport
  wires:
  Position Calculation 1/1(Position) -> Out1/1
  Reset 1/1 -> Position Calculation 1/3(Reset (Impulse))
  Sin && Cos1/1 -> Filters 1/1(Sin && Cos)
  Filters 1/2(Cos) -> Position Calculation 1/2(Cos)
  Filters 1/1(Sin) -> Position Calculation 1/1(Sin)

== system IRP/Const/Subsystem/Position 2 ==
  Sin && Cos2 : Inport
  Reset 2 : Inport  Port=2
  Filters 2 : Subsystem
  Position Calculation 2 : Subsystem
  Out1 : Outport
  wires:
  Position Calculation 2/1(Position) -> Out1/1
  Reset 2/1 -> Position Calculation 2/3(Reset (Impulse))
  Sin && Cos2/1 -> Filters 2/1(Sin && Cos)
  Filters 2/2(Cos) -> Position Calculation 2/2(Cos)
  Filters 2/1(Sin) -> Position Calculation 2/1(Sin)

== system IRP/Const/Subsystem/Position 3 ==
  Sin && Cos3 : Inport
  Reset 3 : Inport  Port=2
  Filters 3 : Subsystem
  Position Calculation 3 : Subsystem
  Out1 : Outport
  wires:
  Position Calculation 3/1(Position) -> Out1/1
  Reset 3/1 -> Position Calculation 3/3(Reset (Impulse))
  Sin && Cos3/1 -> Filters 3/1(Sin && Cos)
  Filters 3/2(Cos) -> Position Calculation 3/2(Cos)
  Filters 3/1(Sin) -> Position Calculation 3/1(Sin)

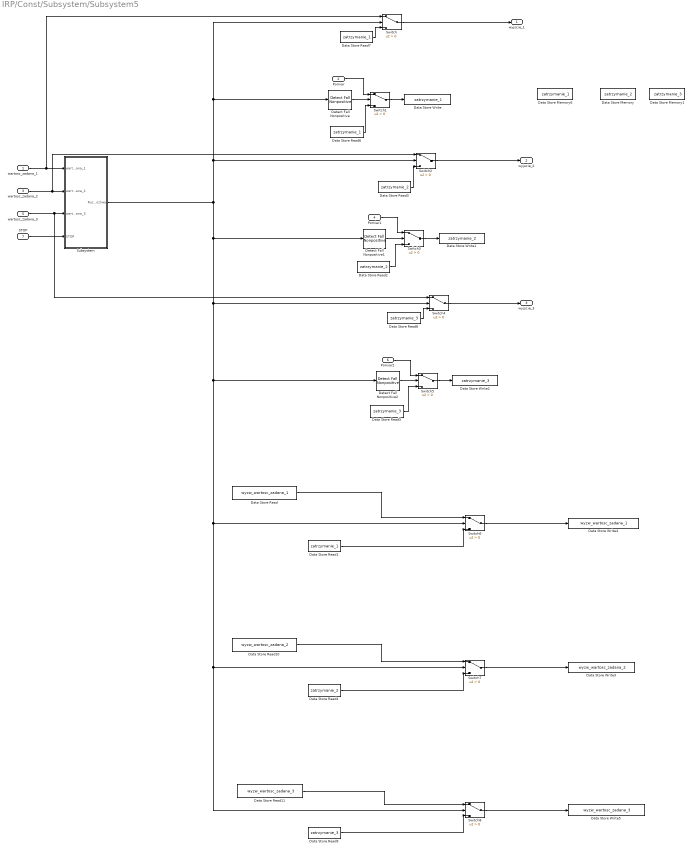
== system IRP/Const/Subsystem/Subsystem5 ==
  wartosc_zadana_1 : Inport
  Pomiar : Inport  Port=2
  wartosc_zadana_2 : Inport  Port=3
  Pomiar1 : Inport  Port=4
  wartosc_zadana_3 : Inport  Port=5
  Pomiar2 : Inport  Port=6
  STOP : Inport  Port=7
  Data Store Memory : DataStoreMemory  DataStoreName=zatrzymanie_2  ReadBeforeWriteMsg=warning  WriteAfterWriteMsg=warning  WriteAfterReadMsg=warning
  Data Store Memory1 : DataStoreMemory  DataStoreName=zatrzymanie_3  ReadBeforeWriteMsg=warning  WriteAfterWriteMsg=warning  WriteAfterReadMsg=warning
  Data Store Memory6 : DataStoreMemory  DataStoreName=zatrzymanie_1  ReadBeforeWriteMsg=warning  WriteAfterWriteMsg=warning  WriteAfterReadMsg=warning
  Data Store Read : DataStoreRead  DataStoreName=wyzw_wartosc_zadana_1
  Data Store Read1 : DataStoreRead  DataStoreName=zatrzymanie_1
  Data Store Read10 : DataStoreRead  DataStoreName=wyzw_wartosc_zadana_2
  Data Store Read11 : DataStoreRead  DataStoreName=wyzw_wartosc_zadana_3
  Data Store Read2 : DataStoreRead  DataStoreName=zatrzymanie_2
  Data Store Read3 : DataStoreRead  DataStoreName=zatrzymanie_2
  Data Store Read4 : DataStoreRead  DataStoreName=zatrzymanie_2
  Data Store Read5 : DataStoreRead  DataStoreName=zatrzymanie_3
  Data Store Read6 : DataStoreRead  DataStoreName=zatrzymanie_1
  Data Store Read7 : DataStoreRead  DataStoreName=zatrzymanie_1
  Data Store Read8 : DataStoreRead  DataStoreName=zatrzymanie_3
  Data Store Read9 : DataStoreRead  DataStoreName=zatrzymanie_3
  Data Store Write : DataStoreWrite  DataStoreName=zatrzymanie_1
  Data Store Write1 : DataStoreWrite  DataStoreName=zatrzymanie_2
  Data Store Write2 : DataStoreWrite  DataStoreName=zatrzymanie_3
  Data Store Write3 : DataStoreWrite  DataStoreName=wyzw_wartosc_zadana_2
  Data Store Write4 : DataStoreWrite  DataStoreName=wyzw_wartosc_zadana_1
  Data Store Write5 : DataStoreWrite  DataStoreName=wyzw_wartosc_zadana_3
  Detect Fall Nonpositive : simulink/Logic and Bit Operations/Detect Fall Nonpositive  vinit=0  InputProcessing=Inherited  OutDataTypeStr=boolean
  Detect Fall Nonpositive1 : simulink/Logic and Bit Operations/Detect Fall Nonpositive  vinit=0  InputProcessing=Inherited  OutDataTypeStr=boolean
  Detect Fall Nonpositive2 : simulink/Logic and Bit Operations/Detect Fall Nonpositive  vinit=0  InputProcessing=Inherited  OutDataTypeStr=boolean
  Subsystem : Subsystem
  Switch{,1..8} (9 alike) : Switch  Criteria=u2 > Threshold
  wyjscie_1 : Outport
  wyjscie_2 : Outport  Port=2
  "wyjscie_3 " : Outport  Port=3
  wires:
  Pomiar/1 -> Switch1/1
  Switch1/1 -> Data Store Write/1
  Data Store Read6/1 -> Switch1/3
  Data Store Read7/1 -> Switch/3
  Switch/1 -> wyjscie_1/1
  Detect Fall Nonpositive/1 -> Switch1/2
  Detect Fall Nonpositive1/1 -> Switch3/2
  Pomiar1/1 -> Switch3/1
  Switch3/1 -> Data Store Write1/1
  Data Store Read2/1 -> Switch3/3
  Data Store Read3/1 -> Switch2/3
  Switch2/1 -> wyjscie_2/1
  Detect Fall Nonpositive2/1 -> Switch5/2
  Pomiar2/1 -> Switch5/1
  Switch5/1 -> Data Store Write2/1
  Data Store Read5/1 -> Switch5/3
  Data Store Read8/1 -> Switch4/3
  Switch4/1 -> "wyjscie_3 "/1
  wartosc_zadana_1/1 -> Switch/1, Subsystem/1(wartosc_zadana_1)
  wartosc_zadana_2/1 -> Switch2/1, Subsystem/2(wartosc_zadana_2)
  wartosc_zadana_3/1 -> Switch4/1, Subsystem/3(wartosc_zadana_3)
  STOP/1 -> Subsystem/4(STOP)
  Data Store Read1/1 -> Switch6/3
  Switch6/1 -> Data Store Write4/1
  Data Store Read/1 -> Switch6/1
  Data Store Read4/1 -> Switch7/3
  Switch7/1 -> Data Store Write3/1
  Data Store Read10/1 -> Switch7/1
  Subsystem/1(Ruch_mozliwy) -> Switch4/2, Switch8/2, Switch7/2, Switch6/2, Detect Fall Nonpositive2/1, Detect Fall Nonpositive1/1, Switch2/2, Switch/2, Detect Fall Nonpositive/1
  Data Store Read9/1 -> Switch8/3
  Switch8/1 -> Data Store Write5/1
  Data Store Read11/1 -> Switch8/1

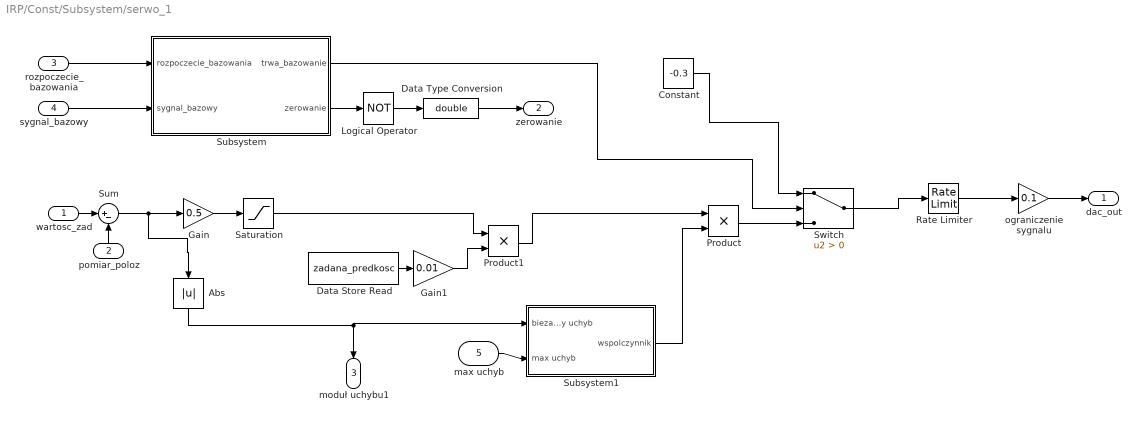
== system IRP/Const/Subsystem/serwo_1 ==
  wartosc_zad : Inport
  pomiar_poloz : Inport  Port=2
  rozpoczecie_bazowania : Inport  Port=3
  sygnal_bazowy : Inport  Port=4
  max uchyb : Inport  Port=5
  Abs : Abs
  Constant : Constant  Value=-0.3
  Data Store Read : DataStoreRead  DataStoreName=zadana_predkosc
  Data Type Conversion : DataTypeConversion  OutDataTypeStr=double
  Gain : Gain  Gain=0.5
  Gain1 : Gain  Gain=0.01
  Logical Operator : Logic  Operator=NOT  AllPortsSameDT=off  OutDataTypeStr=boolean
  Product : Product
  Product1 : Product
  Rate Limiter : RateLimiter  RisingSlewLimit=50  FallingSlewLimit=-50  SampleTimeMode=inherited
  Saturation : Saturate  UpperLimit=3  LowerLimit=-3
  Subsystem : Subsystem
  Subsystem1 : Subsystem
  Sum : Sum  Inputs=|+-
  Switch : Switch  Criteria=u2 > Threshold
  ograniczenie sygnalu : Gain  Gain=0.1
  dac_out : Outport
  zerowanie : Outport  Port=2
  moduł uchybu1 : Outport  Port=3
  wires:
  pomiar_poloz/1 -> Sum/2
  wartosc_zad/1 -> Sum/1
  Gain/1 -> Saturation/1
  Sum/1 -> Abs/1, Gain/1
  Rate Limiter/1 -> ograniczenie sygnalu/1
  ograniczenie sygnalu/1 -> dac_out/1
  Constant/1 -> Switch/1
  Subsystem/1(trwa_bazowanie) -> Switch/2
  Subsystem/2(zerowanie) -> Logical Operator/1
  Logical Operator/1 -> Data Type Conversion/1
  Data Type Conversion/1 -> zerowanie/1
  rozpoczecie_bazowania/1 -> Subsystem/1(rozpoczecie_bazowania)
  sygnal_bazowy/1 -> Subsystem/2(sygnal_bazowy)
  Switch/1 -> Rate Limiter/1
  Abs/1 -> moduł uchybu1/1, Subsystem1/1(biezacy uchyb)
  max uchyb/1 -> Subsystem1/2(max uchyb)
  Product/1 -> Switch/3
  Subsystem1/1(wspolczynnik) -> Product/2
  Saturation/1 -> Product1/1
  Product1/1 -> Product/1
  Data Store Read/1 -> Gain1/1
  Gain1/1 -> Product1/2

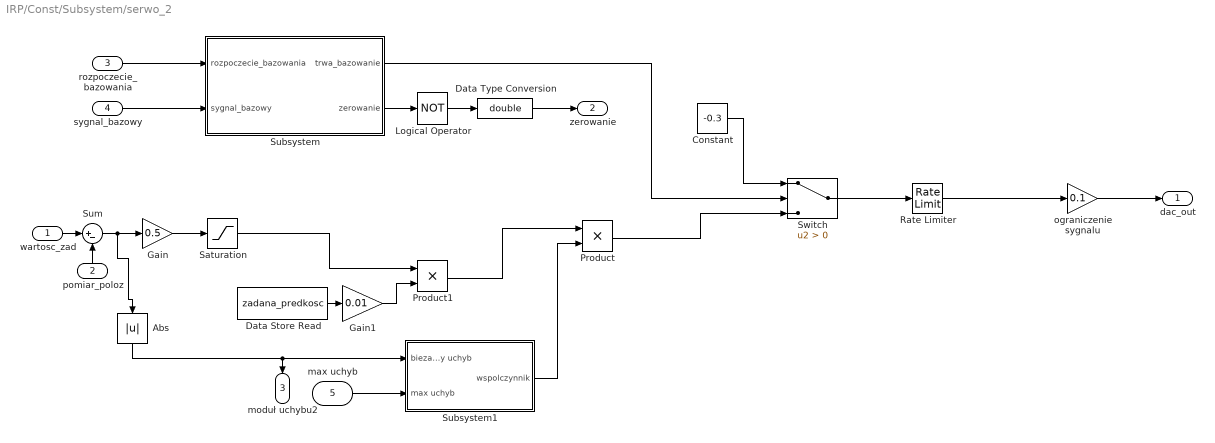
== system IRP/Const/Subsystem/serwo_2 ==
  wartosc_zad : Inport
  pomiar_poloz : Inport  Port=2
  rozpoczecie_bazowania : Inport  Port=3
  sygnal_bazowy : Inport  Port=4
  max uchyb : Inport  Port=5
  Abs : Abs
  Constant : Constant  Value=-0.3
  Data Store Read : DataStoreRead  DataStoreName=zadana_predkosc
  Data Type Conversion : DataTypeConversion  OutDataTypeStr=double
  Gain : Gain  Gain=0.5
  Gain1 : Gain  Gain=0.01
  Logical Operator : Logic  Operator=NOT  AllPortsSameDT=off  OutDataTypeStr=boolean
  Product : Product
  Product1 : Product
  Rate Limiter : RateLimiter  RisingSlewLimit=50  FallingSlewLimit=-50  SampleTimeMode=inherited
  Saturation : Saturate  UpperLimit=3  LowerLimit=-3
  Subsystem : Subsystem
  Subsystem1 : Subsystem
  Sum : Sum  Inputs=|+-
  Switch : Switch  Criteria=u2 > Threshold
  ograniczenie sygnalu : Gain  Gain=0.1
  dac_out : Outport
  zerowanie : Outport  Port=2
  moduł uchybu2 : Outport  Port=3
  wires:
  pomiar_poloz/1 -> Sum/2
  wartosc_zad/1 -> Sum/1
  Gain/1 -> Saturation/1
  Rate Limiter/1 -> ograniczenie sygnalu/1
  ograniczenie sygnalu/1 -> dac_out/1
  Constant/1 -> Switch/1
  Subsystem/1(trwa_bazowanie) -> Switch/2
  Subsystem/2(zerowanie) -> Logical Operator/1
  Logical Operator/1 -> Data Type Conversion/1
  Data Type Conversion/1 -> zerowanie/1
  rozpoczecie_bazowania/1 -> Subsystem/1(rozpoczecie_bazowania)
  sygnal_bazowy/1 -> Subsystem/2(sygnal_bazowy)
  Switch/1 -> Rate Limiter/1
  Sum/1 -> Abs/1, Gain/1
  Abs/1 -> Subsystem1/1(biezacy uchyb), moduł uchybu2/1
  max uchyb/1 -> Subsystem1/2(max uchyb)
  Subsystem1/1(wspolczynnik) -> Product/2
  Product/1 -> Switch/3
  Saturation/1 -> Product1/1
  Product1/1 -> Product/1
  Data Store Read/1 -> Gain1/1
  Gain1/1 -> Product1/2

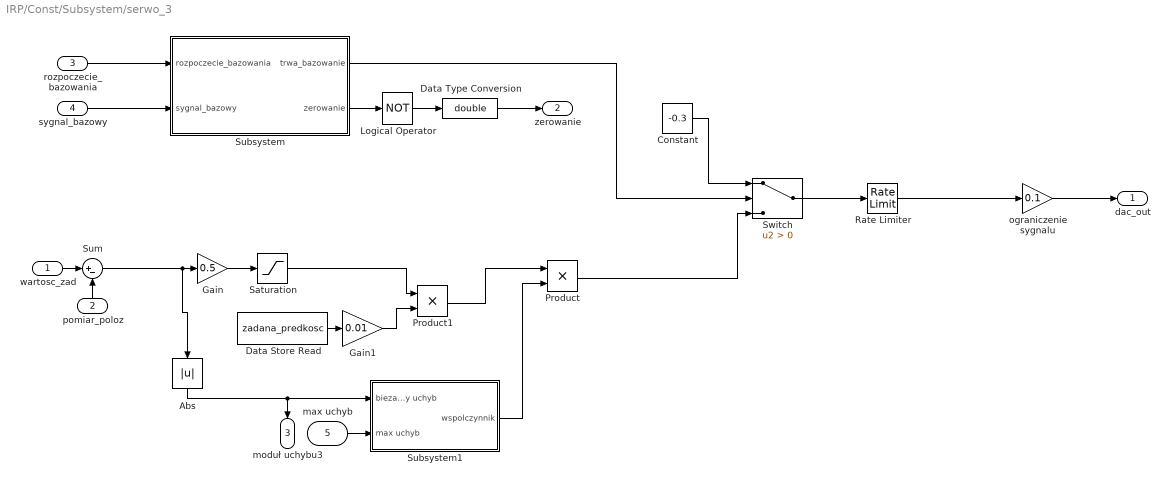
== system IRP/Const/Subsystem/serwo_3 ==
  wartosc_zad : Inport
  pomiar_poloz : Inport  Port=2
  rozpoczecie_bazowania : Inport  Port=3
  sygnal_bazowy : Inport  Port=4
  max uchyb : Inport  Port=5
  Abs : Abs
  Constant : Constant  Value=-0.3
  Data Store Read : DataStoreRead  DataStoreName=zadana_predkosc
  Data Type Conversion : DataTypeConversion  OutDataTypeStr=double
  Gain : Gain  Gain=0.5
  Gain1 : Gain  Gain=0.01
  Logical Operator : Logic  Operator=NOT  AllPortsSameDT=off  OutDataTypeStr=boolean
  Product : Product
  Product1 : Product
  Rate Limiter : RateLimiter  RisingSlewLimit=50  FallingSlewLimit=-50  SampleTimeMode=inherited
  Saturation : Saturate  UpperLimit=3  LowerLimit=-3
  Subsystem : Subsystem
  Subsystem1 : Subsystem
  Sum : Sum  Inputs=|+-
  Switch : Switch  Criteria=u2 > Threshold
  ograniczenie sygnalu : Gain  Gain=0.1
  dac_out : Outport
  zerowanie : Outport  Port=2
  moduł uchybu3 : Outport  Port=3
  wires:
  pomiar_poloz/1 -> Sum/2
  wartosc_zad/1 -> Sum/1
  Gain/1 -> Saturation/1
  Rate Limiter/1 -> ograniczenie sygnalu/1
  ograniczenie sygnalu/1 -> dac_out/1
  Constant/1 -> Switch/1
  Subsystem/1(trwa_bazowanie) -> Switch/2
  Subsystem/2(zerowanie) -> Logical Operator/1
  Logical Operator/1 -> Data Type Conversion/1
  Data Type Conversion/1 -> zerowanie/1
  rozpoczecie_bazowania/1 -> Subsystem/1(rozpoczecie_bazowania)
  sygnal_bazowy/1 -> Subsystem/2(sygnal_bazowy)
  Switch/1 -> Rate Limiter/1
  Sum/1 -> Abs/1, Gain/1
  Abs/1 -> Subsystem1/1(biezacy uchyb), moduł uchybu3/1
  Subsystem1/1(wspolczynnik) -> Product/2
  Product/1 -> Switch/3
  max uchyb/1 -> Subsystem1/2(max uchyb)
  Saturation/1 -> Product1/1
  Product1/1 -> Product/1
  Data Store Read/1 -> Gain1/1
  Gain1/1 -> Product1/2

== system IRP/Const/Subsystem/serwo_4_5 ==
  In1 : Inport
  In3 : Inport  Port=2
  Constant : Constant
  Data Store Memory1 : DataStoreMemory  DataStoreName=Wartosc_zad_4  ReadBeforeWriteMsg=warning  WriteAfterWriteMsg=warning  WriteAfterReadMsg=warning
  Data Store Memory2 : DataStoreMemory  DataStoreName=Wartosc_zad_5  ReadBeforeWriteMsg=warning  WriteAfterWriteMsg=warning  WriteAfterReadMsg=warning
  Data Store Read4 : DataStoreRead  DataStoreName=Wartosc_zad_4
  Data Store Read5 : DataStoreRead  DataStoreName=Wartosc_zad_5
  Position 4 : Subsystem
  Position 5 : Subsystem
  serwo_4 : Subsystem
  serwo_5 : Subsystem
  Out1 : Outport
  Out2 : Outport  Port=2
  wires:
  In1/1 -> Position 4/1(Sin && Cos4)
  In3/1 -> Position 5/1(Sin && Cos5)
  Data Store Read4/1 -> serwo_4/1(wartosc_zad)
  Data Store Read5/1 -> serwo_5/1(wartosc_zad)
  Position 4/1(Out1) -> serwo_4/2(pomiar_poloz)
  Position 5/1(Out1) -> serwo_5/2(pomiar_poloz)
  serwo_4/1(dac_out) -> Out1/1
  serwo_5/1(dac_out) -> Out2/1
  Constant/1 -> Position 5/2(Reset 5), Position 4/2(Reset 4)

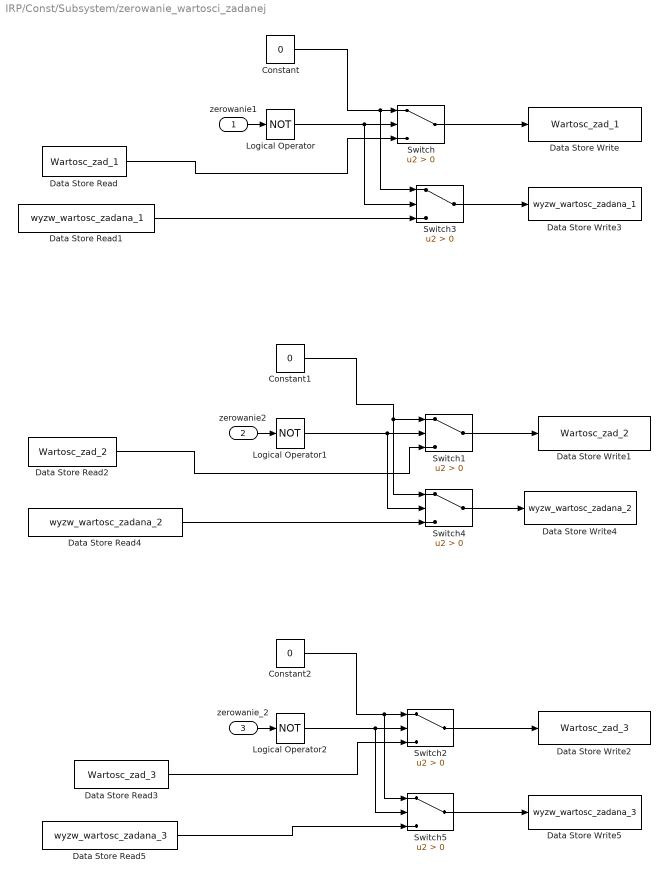
== system IRP/Const/Subsystem/zerowanie_wartosci_zadanej ==
  zerowanie1 : Inport
  zerowanie2 : Inport  Port=2
  zerowanie_2 : Inport  Port=3
  Constant : Constant  Value=0
  Constant1 : Constant  Value=0
  Constant2 : Constant  Value=0
  Data Store Read : DataStoreRead  DataStoreName=Wartosc_zad_1
  Data Store Read1 : DataStoreRead  DataStoreName=wyzw_wartosc_zadana_1
  Data Store Read2 : DataStoreRead  DataStoreName=Wartosc_zad_2
  Data Store Read3 : DataStoreRead  DataStoreName=Wartosc_zad_3
  Data Store Read4 : DataStoreRead  DataStoreName=wyzw_wartosc_zadana_2
  Data Store Read5 : DataStoreRead  DataStoreName=wyzw_wartosc_zadana_3
  Data Store Write : DataStoreWrite  DataStoreName=Wartosc_zad_1
  Data Store Write1 : DataStoreWrite  DataStoreName=Wartosc_zad_2
  Data Store Write2 : DataStoreWrite  DataStoreName=Wartosc_zad_3
  Data Store Write3 : DataStoreWrite  DataStoreName=wyzw_wartosc_zadana_1
  Data Store Write4 : DataStoreWrite  DataStoreName=wyzw_wartosc_zadana_2
  Data Store Write5 : DataStoreWrite  DataStoreName=wyzw_wartosc_zadana_3
  Logical Operator : Logic  Operator=NOT  AllPortsSameDT=off  OutDataTypeStr=boolean
  Logical Operator1 : Logic  Operator=NOT  AllPortsSameDT=off  OutDataTypeStr=boolean
  Logical Operator2 : Logic  Operator=NOT  AllPortsSameDT=off  OutDataTypeStr=boolean
  Switch{,1..5} (6 alike) : Switch  Criteria=u2 > Threshold
  wires:
  Constant/1 -> Switch3/1, Switch/1
  zerowanie1/1 -> Logical Operator/1
  Constant1/1 -> Switch4/1, Switch1/1
  Logical Operator1/1 -> Switch4/2, Switch1/2
  zerowanie2/1 -> Logical Operator1/1
  Logical Operator2/1 -> Switch5/2, Switch2/2
  zerowanie_2/1 -> Logical Operator2/1
  Switch/1 -> Data Store Write/1
  Switch1/1 -> Data Store Write1/1
  Switch2/1 -> Data Store Write2/1
  Data Store Read/1 -> Switch/3
  Data Store Read2/1 -> Switch1/3
  Data Store Read3/1 -> Switch2/3
  Logical Operator/1 -> Switch3/2, Switch/2
  Data Store Read1/1 -> Switch3/3
  Data Store Read4/1 -> Switch4/3
  Constant2/1 -> Switch5/1, Switch2/1
  Data Store Read5/1 -> Switch5/3
  Switch4/1 -> Data Store Write4/1
  Switch5/1 -> Data Store Write5/1
  Switch3/1 -> Data Store Write3/1

== system IRP/Const/Subsystem1/Subsystem ==
  fi1 : Inport
  fi2 : Inport  Port=2
  fi3 : Inport  Port=3
  p2 : Inport  Port=4
  p3 : Inport  Port=5
  Add : Sum
  Product : Product
  Product1 : Product
  Product2 : Product
  Trigonometric Function : Trigonometry  Operator=cos
  Trigonometric Function1 : Trigonometry
  Trigonometric Function2 : Trigonometry  Operator=cos
  x : Outport
  wires:
  fi1/1 -> Trigonometric Function/1
  Trigonometric Function/1 -> Product2/1
  Product2/1 -> x/1
  Add/1 -> Product2/2
  Product/1 -> Add/1
  Product1/1 -> Add/2
  Trigonometric Function1/1 -> Product/1
  fi2/1 -> Trigonometric Function1/1
  p2/1 -> Product/2
  fi3/1 -> Trigonometric Function2/1
  Trigonometric Function2/1 -> Product1/1
  p3/1 -> Product1/2

== system IRP/Const/Subsystem1/Subsystem1 ==
  fi1 : Inport
  fi2 : Inport  Port=2
  fi3 : Inport  Port=3
  p2 : Inport  Port=4
  p3 : Inport  Port=5
  Add : Sum
  Product : Product
  Product1 : Product
  Product2 : Product
  Trigonometric Function : Trigonometry
  Trigonometric Function1 : Trigonometry
  Trigonometric Function2 : Trigonometry  Operator=cos
  y : Outport
  wires:
  fi1/1 -> Trigonometric Function/1
  Trigonometric Function/1 -> Product2/1
  Product2/1 -> y/1
  Add/1 -> Product2/2
  Product/1 -> Add/1
  Product1/1 -> Add/2
  Trigonometric Function1/1 -> Product/1
  fi2/1 -> Trigonometric Function1/1
  p2/1 -> Product/2
  fi3/1 -> Trigonometric Function2/1
  Trigonometric Function2/1 -> Product1/1
  p3/1 -> Product1/2

== system IRP/Const/Subsystem1/Subsystem2 ==
  p1 : Inport
  fi2 : Inport  Port=2
  fi3 : Inport  Port=3
  p2 : Inport  Port=4
  p3 : Inport  Port=5
  Add : Sum  Inputs=++-
  Product : Product
  Product1 : Product
  Trigonometric Function1 : Trigonometry  Operator=cos
  Trigonometric Function2 : Trigonometry
  z : Outport
  wires:
  p1/1 -> Add/1
  Trigonometric Function1/1 -> Product/1
  fi2/1 -> Trigonometric Function1/1
  p2/1 -> Product/2
  fi3/1 -> Trigonometric Function2/1
  Trigonometric Function2/1 -> Product1/1
  p3/1 -> Product1/2
  Add/1 -> z/1
  Product/1 -> Add/2
  Product1/1 -> Add/3

== system IRP/Input/Logic /Subsystem ==
  In1 : Inport
  Gain : Gain  Gain=-1
  Logical Operator : Logic  AllPortsSameDT=off
  Switch1 : Switch  Criteria=u2 > Threshold  Threshold=-160
  Switch2 : Switch  Criteria=u2 > Threshold  Threshold=-160
  "logic0 " : Constant  Value=0
  "logic1 " : Constant
  Out1 : Outport
  wires:
  Logical Operator/1 -> Out1/1
  Switch1/1 -> Logical Operator/1
  "logic0 "/1 -> Switch1/3, Switch2/3
  In1/1 -> Gain/1, Switch1/2
  Switch2/1 -> Logical Operator/2
  Gain/1 -> Switch2/2
  "logic1 "/1 -> Switch2/1, Switch1/1

== system IRP/Input/Logic /Subsystem1 ==
  In1 : Inport
  Gain : Gain  Gain=-1
  Logical Operator : Logic  AllPortsSameDT=off
  Switch1 : Switch  Criteria=u2 > Threshold  Threshold=-40
  Switch2 : Switch  Criteria=u2 > Threshold  Threshold=-40
  "logic0 " : Constant  Value=0
  "logic1 " : Constant
  Out1 : Outport
  wires:
  Logical Operator/1 -> Out1/1
  Switch1/1 -> Logical Operator/1
  "logic0 "/1 -> Switch1/3, Switch2/3
  In1/1 -> Gain/1, Switch1/2
  Switch2/1 -> Logical Operator/2
  Gain/1 -> Switch2/2
  "logic1 "/1 -> Switch2/1, Switch1/1

== system IRP/Input/Logic /Subsystem2 ==
  In1 : Inport
  Gain : Gain  Gain=-1
  Logical Operator : Logic  AllPortsSameDT=off
  Switch1 : Switch  Criteria=u2 > Threshold  Threshold=-25
  Switch2 : Switch  Criteria=u2 > Threshold  Threshold=-40
  "logic0 " : Constant  Value=0
  "logic1 " : Constant
  Out1 : Outport
  wires:
  Logical Operator/1 -> Out1/1
  Switch1/1 -> Logical Operator/1
  "logic0 "/1 -> Switch1/3, Switch2/3
  In1/1 -> Gain/1, Switch1/2
  Switch2/1 -> Logical Operator/2
  Gain/1 -> Switch2/2
  "logic1 "/1 -> Switch2/1, Switch1/1

== system IRP/Input/Logic /Subsystem3 ==
  In1 : Inport
  Gain : Gain  Gain=-1
  Logical Operator : Logic  AllPortsSameDT=off
  Switch1 : Switch  Criteria=u2 > Threshold  Threshold=-25
  Switch2 : Switch  Criteria=u2 > Threshold  Threshold=-120
  "logic0 " : Constant  Value=0
  "logic1 " : Constant
  Out1 : Outport
  wires:
  Logical Operator/1 -> Out1/1
  Switch1/1 -> Logical Operator/1
  "logic0 "/1 -> Switch1/3, Switch2/3
  In1/1 -> Gain/1, Switch1/2
  Switch2/1 -> Logical Operator/2
  Gain/1 -> Switch2/2
  "logic1 "/1 -> Switch2/1, Switch1/1

== system IRP/Input/Logic /Subsystem4 ==
  In1 : Inport
  Gain : Gain  Gain=-1
  Logical Operator : Logic  AllPortsSameDT=off
  Switch1 : Switch  Criteria=u2 > Threshold  Threshold=-25
  Switch2 : Switch  Criteria=u2 > Threshold  Threshold=-150
  "logic0 " : Constant  Value=0
  "logic1 " : Constant
  Out1 : Outport
  wires:
  Logical Operator/1 -> Out1/1
  Switch1/1 -> Logical Operator/1
  "logic0 "/1 -> Switch1/3, Switch2/3
  In1/1 -> Gain/1, Switch1/2
  Switch2/1 -> Logical Operator/2
  Gain/1 -> Switch2/2
  "logic1 "/1 -> Switch2/1, Switch1/1
